simulink library "gravity_lib_2"  (R2016b)
settings: Solver=VariableStepAuto  StartTime=0.0  StopTime=10.0  RelTol=1e-3
undefined symbols (not defined in the file or in its folder): sim_params
libraries: aerolibutil x1, aerolibgravity2 x1, gravity_field_lib x1
settings Model: Creator=taylorreynolds  LastModifiedBy=taylorreynolds

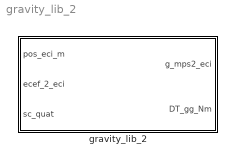
== system gravity_lib_2 ==
  gravity_lib_2 : Subsystem

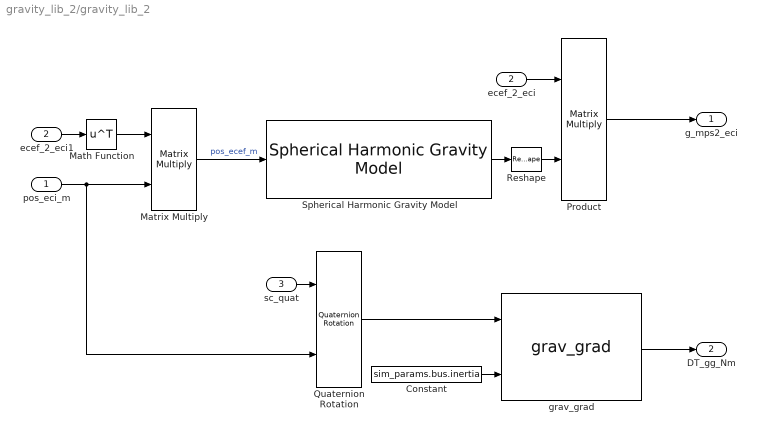
== system gravity_lib_2/gravity_lib_2 ==
  pos_eci_m : Inport
  ecef_2_eci : Inport  Port=2
  sc_quat : Inport  Port=3
  Constant : Constant  Value=sim_params.bus.inertia
  Math Function : Math  Operator=transpose  SaturateOnIntegerOverflow=on
  Matrix Multiply : Product  Multiplication=Matrix(*)
  Product : Product  Multiplication=Matrix(*)
  Quaternion Rotation : aerolibutil/Quaternion Rotation
  Reshape : Reshape  OutputDimensionality=Customize  OutputDimensions=3
  Spherical Harmonic Gravity Model : aerolibgravity2/Spherical Harmonic Gravity Model  units=Metric (MKS)  degree=120  action=Warning  ptype=EGM2008  datafile='aerogmm2b.mat'
  ecef_2_eci1 : InportShadow  Port=2
  grav_grad : gravity_field_lib/grav_dist/grav_grad
  g_mps2_eci : Outport
  DT_gg_Nm : Outport  Port=2
  wires:
  Spherical Harmonic Gravity Model/1 -> Reshape/1
  ecef_2_eci/1 -> Product/1
  Product/1 -> g_mps2_eci/1
  ecef_2_eci1/1 -> Math Function/1
  sc_quat/1 -> Quaternion Rotation/1
  Matrix Multiply/1 -> Spherical Harmonic Gravity Model/1  "pos_ecef_m"
  pos_eci_m/1 -> Quaternion Rotation/2, Matrix Multiply/2
  Quaternion Rotation/1 -> grav_grad/1
  Constant/1 -> grav_grad/2
  grav_grad/1 -> DT_gg_Nm/1
  Math Function/1 -> Matrix Multiply/1
  Reshape/1 -> Product/2
